simulink model "DPT"  (R2023a)
settings: Solver=VariableStepAuto  StartTime=0.0  StopTime=10.0  RelTol=1e-3
values from neighbouring files (symbols this model uses):
  Ja = 7e-6    (= 7e-06)    [init.m]
  K1 = Cm*Cw    (= 4.095)    [init.m]
  T = (Lov+Lya)/Rya    (= 0.0035)    [init.m]
  Uu = 2    [init.m]
settings Model: Creator=Алексей  LastModifiedBy=Алексей

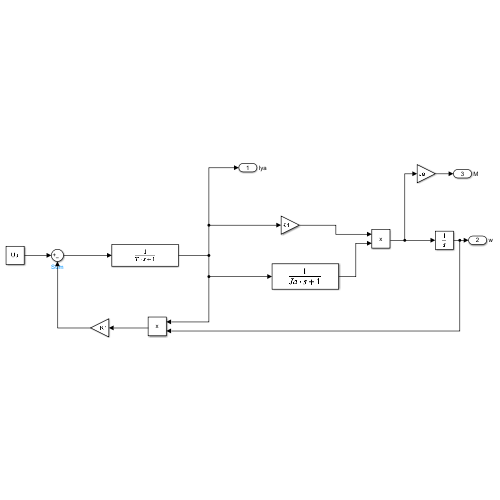
[thumbnail: Simulink's stored preview of the top-level diagram]
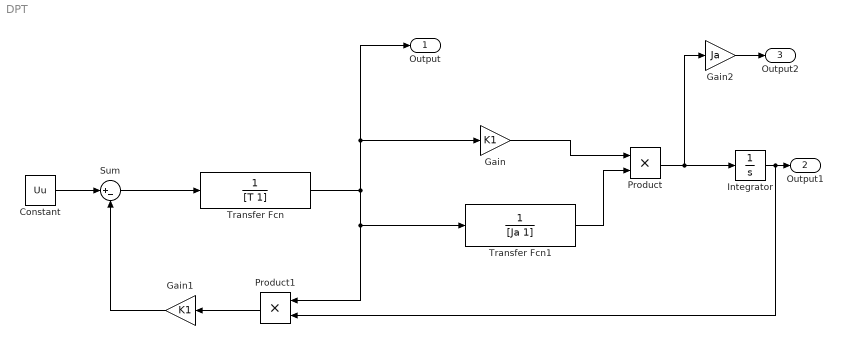
== system DPT ==
  Constant : Constant  Value=Uu
  Gain : Gain  Gain=K1
  Gain1 : Gain  Gain=K1
  Gain2 : Gain  Gain=Ja
  Integrator : Integrator
  Product : Product
  Product1 : Product
  Sum : Sum  Inputs=|+-
  Transfer Fcn : TransferFcn  Denominator=[T 1]
  Transfer Fcn1 : TransferFcn  Denominator=[Ja 1]
  Output : Outport  SignalName=Iya
  Output1 : Outport  Port=2  SignalName=w
  Output2 : Outport  Port=3  SignalName=M
  wires:
  Constant/1 -> Sum/1
  Sum/1 -> Transfer Fcn/1
  Transfer Fcn/1 -> Gain/1, Output/1, Product1/1, Transfer Fcn1/1
  Transfer Fcn1/1 -> Product/2
  Gain/1 -> Product/1
  Product1/1 -> Gain1/1
  Gain1/1 -> Sum/2
  Product/1 -> Gain2/1, Integrator/1
  Integrator/1 -> Product1/2, Output1/1
  Gain2/1 -> Output2/1
